simulink model "PT3_mod"  (R2018b)
settings: Solver=FixedStepAuto  StartTime=0.0  StopTime=tstop  FixedStep=dt  RelTol=1e-3
values from neighbouring files (symbols this model uses):
  a1 = R*C1    (= 0.05185)    [PT3_dat.m]
  a2 = L*(C1+C2)    (= 0.000408)    [PT3_dat.m]
  a3 = R*L*C1*C2    (= 1.23403e-05)    [PT3_dat.m]
  tstep = 1e-6    (= 1e-06)    [PT3_dat.m]
  Uemax = 10    [PT3_dat.m]
settings Model: Creator=Peter  LastModifiedBy=Peter

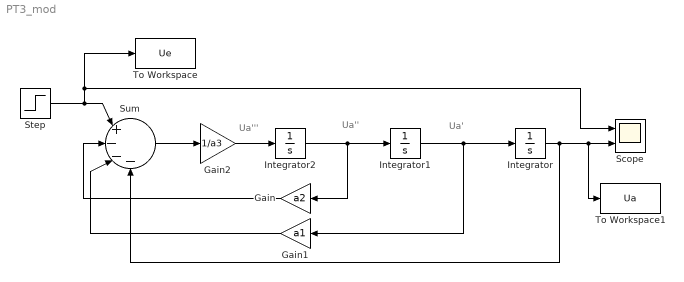
== system PT3_mod ==
  note: Ua'
  note: Ua''
  note: Ua'''
  Gain : Gain  Gain=a2
  Gain1 : Gain  Gain=a1
  Gain2 : Gain  Gain=1/a3
  Integrator : Integrator
  Integrator1 : Integrator
  Integrator2 : Integrator
  Scope : Scope  NumInputPorts=2
  Step : Step  Time=tstep  After=Uemax  SampleTime=0
  Sum : Sum  Inputs=|+---
  To Workspace : ToWorkspace  VariableName=Ue  SampleTime=-1
  To Workspace1 : ToWorkspace  VariableName=Ua  SampleTime=-1
  wires:
  Integrator2/1 -> Gain/1, Integrator1/1
  Integrator1/1 -> Gain1/1, Integrator/1
  Step/1 -> Scope/1, To Workspace/1, Sum/1
  Gain/1 -> Sum/2
  Gain1/1 -> Sum/3
  Integrator/1 -> Sum/4, To Workspace1/1, Scope/2
  Sum/1 -> Gain2/1
  Gain2/1 -> Integrator2/1
